simulink model "pendule_inverse"  (R2023a)
settings: Solver=ode1  StartTime=0.0  StopTime=10.0  RelTol=1e-3
undefined symbols (not defined in the file): g, K, l, ue, x0, xe
settings Model: Creator=fhudrisi  LastModifiedBy=gwr2526
settings OptimizationCC: ReuseModelBlockBuffer=off
settings DebuggingCC: AlgebraicLoopMsg=none  UnconnectedInputMsg=warning  UnconnectedOutputMsg=warning  UnconnectedLineMsg=warning
settings ModelReferenceCC: EnableRefExpFcnMdlSchedulingChecks=on
settings RTWCC: DLArmComputeVersion=19.05

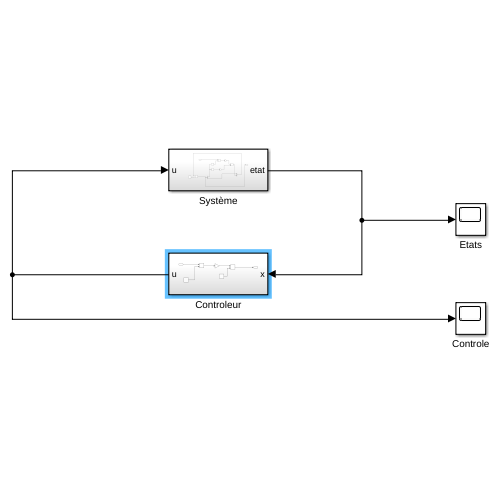
[thumbnail: Simulink's stored preview of the top-level diagram]
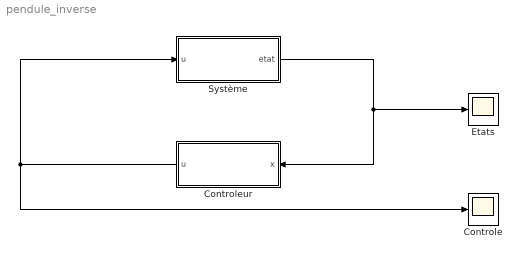
== system pendule_inverse ==
  Controle : Scope
  Controleur : Subsystem
  Etats : Scope
  Système : Subsystem
  wires:
  Système/1(etat) -> Controleur/1(x), Etats/1
  Controleur/1(u) -> Système/1(u), Controle/1

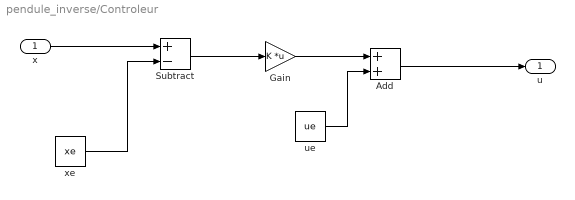
== system pendule_inverse/Controleur ==
  x : Inport
  Add : Sum
  Gain : Gain  Gain=K  Multiplication=Matrix(K*u)
  Subtract : Sum  Inputs=+-
  ue : Constant  Value=ue
  xe : Constant  Value=xe
  u : Outport
  wires:
  Add/1 -> u/1
  Subtract/1 -> Gain/1
  x/1 -> Subtract/1
  ue/1 -> Add/2
  Gain/1 -> Add/1
  xe/1 -> Subtract/2

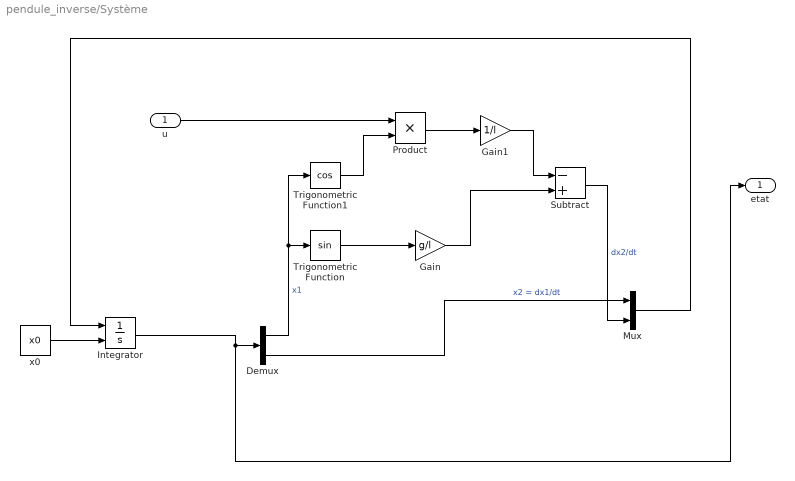
== system pendule_inverse/Système ==
  u : Inport
  Demux : Demux  Outputs=2
  Gain : Gain  Gain=g/l
  Gain1 : Gain  Gain=1/l
  Integrator : Integrator  InitialConditionSource=external
  Mux : Mux  Inputs=2
  Product : Product
  Subtract : Sum  Inputs=-+
  Trigonometric Function : Trigonometry
  Trigonometric Function1 : Trigonometry  Operator=cos
  x0 : Constant  Value=x0
  etat : Outport
  wires:
  Demux/1 -> Trigonometric Function1/1, Trigonometric Function/1  "x1"
  Demux/2 -> Mux/1  "x2 = dx1/dt"
  Trigonometric Function1/1 -> Product/2
  Integrator/1 -> etat/1, Demux/1
  Gain/1 -> Subtract/2
  Subtract/1 -> Mux/2  "dx2/dt"
  Trigonometric Function/1 -> Gain/1
  u/1 -> Product/1
  Product/1 -> Gain1/1
  Gain1/1 -> Subtract/1
  Mux/1 -> Integrator/1
  x0/1 -> Integrator/2
